simulink model "VFlexP"  (R2025a)
settings: Solver=ode23tb  StartTime=0.0  StopTime=40  FixedStep=5e-5
model workspace (MAT data in the model file):
  DCop_DCBUCK : object (value not decoded)
  Grid_CCVSC_idx = [2; 3; 4; 5; 6; 7; 8; 9; 10; 11; 12]
  Grid_CCVSCs = 1
  Grid_CCVSCs_buses = 1
  Grid_CCVSCs_toM = [0 1 0 0 0 0 0 0 0 0 0 0 ... (781 elements, 71x11)]
  Grid_C_Lines = [0.1 0.1 0.1 0.1]
  Grid_Cbuses = [0.05000002 0.10000002 0.10000002 0.10000002 0.05000002]
  Grid_DC : object (value not decoded)
  Grid_DCop_DCBUCK : object (value not decoded)
  Grid_DCop_DC_PES : object (value not decoded)
  Grid_DFIGs = 1
  Grid_DFIGs_buses = 1
  Grid_DGs : string (value not decoded)
  Grid_From_buses = [1 2 4 4]
  Grid_GFls = 1
  Grid_GFls_buses = 1
  Grid_GFr_idx = [1; 2; 3]
  Grid_GFrs = 1
  Grid_GFrs_buses = 1
  Grid_GFrs_toM = [1 0 0 0 0 0 0 0 0 1 0 0 ... (15 elements, 5x3)]
  Grid_IG_idx = 1
  Grid_IGs = 1
  Grid_IGs_buses = 1
  Grid_IGs_toM = [1; 0]
  Grid_L_Lines = [0.5 0.5 0.5 0.5]
  Grid_L_Loads = [0.000959999944704 0.000156249997559 0.00154855477548]
  Grid_Lines_fromM : object (value not decoded)
  Grid_Lines_toM : object (value not decoded)
  Grid_Load_buses = [2; 3; 4]
  Grid_Load_busesDC = []
  Grid_MGES_idx = [1; 2; 3]
  Grid_MGESs = 1
  Grid_MGESs_buses = [1; 5; 3]
  Grid_MGESs_toM = [1 0 0 0 0 0 0 0 0 1 0 0 ... (15 elements, 5x3)]
  Grid_MSGs = 1
  Grid_MSGs_buses = 1
  Grid_Nbuses = 5
  Grid_PQ_gen = [3; 2; 2]
  Grid_Ploads = [1250 4000 1250]
  Grid_PloadsDC = []
  Grid_Ps_lf = [0.274439537683 0.78 0.3]
  Grid_Qloads = [0.3 0.5 0.5]
  Grid_Qs_lf = [-0.0366071562958 0.126505596722 -0.0162964024532]
  Grid_R_Lines = [0.01 0.01 0.01 0.01]
  Grid_R_Loads = [3.9999997696 1.24999998047 3.8713869387]
  Grid_R_Loads_DC = 0
  Grid_Rcf = [50000000 50000000 50000000 50000000 50000000]
  Grid_SCs = 1
  Grid_SCs_buses = 1
  Grid_SG_idx = 1
  Grid_SGs = 1
  Grid_SGs_buses = 1
  Grid_SGs_toM = [1; 0]
  Grid_To_buses = [2 3 3 5]
  Grid_VCVSC_idx = [1; 2; 3; 4; 5; 6; 7; 8; 9; 10; 11; 12]
  Grid_VCVSCs = 1
  Grid_VCVSCs_buses = [1; 2; 3; 6; 8; 9; 12; 58; 59; 60; 63; 65]
  Grid_VCVSCs_toM = [1 0 0 0 0 0 0 0 0 0 0 0 ... (852 elements, 71x12)]
  Grid_VSM_idx = [1; 2; 3]
  Grid_VSMs = 1
  Grid_VSMs_buses = 1
  Grid_VSMs_toM = [1 0 0 0 0 0 0 0 0 1 0 0 ... (15 elements, 5x3)]
  Grid_admitt_matrix = [2.15353135314-19.7953135314i  -1.9801980198+19.801980198i; -1.9801980198+19.801980198i  2.15353135314-19.7953135314i]
  Grid_admitt_matrix_noloads = [1.98686468647-19.7953135314i  -1.9801980198+19.801980198i; -1.9801980198+19.801980198i  1.98686468647-19.7953135314i]
  Grid_bus = [1; 2; 6; 7; 8]
  Grid_busDC_complexity = [1 1 1]
  Grid_busDC_complexity_PF = [2 2 2]
  Grid_bus_complexity = [1 1 1 1 1]
  Grid_bus_complexity_PF = [1 1 1 1 1]
  Grid_buses_lf = [1; 5; 3]
  Grid_conductance_matrix = [100.00000002  -100  0; -100  200.00000002  -100; 0  -100  100.00000002]
  Grid_conductance_matrix_noloads = [100.00000002  -100  0; -100  200.00000002  -100; 0  -100  100.00000002]
  Grid_fref : object (value not decoded)
  Grid_gen_static_params : mBase (value not decoded)
  Grid_iPs_lf = [3.64378984326 1.28205128205 3.33333333333]
  Grid_iQs_lf = [-27.3170631425 7.90478860943 -61.3632366329]
  Grid_iadmitt_matrix = [2.88165849328-0.0982918688642i  2.87905051706-0.123273862303i; 2.87905051706-0.123273862303i  2.88165849328-0.0982918688642i]
  Grid_iadmitt_matrix_noloads = [37.5012524798-37.4874983544i  37.4987475202-37.5125016456i; 37.4987475202-37.5125016456i  37.5012524798-37.4874983544i]
  Grid_iconductance_matrix = [16666671.4556  16666671.4489  16666671.4456; 16666671.4489  16666671.4522  16666671.4489; 16666671.4456  16666671.4489  16666671.4556]
  Grid_iconductance_matrix_noloads = [16666671.4556  16666671.4489  16666671.4456; 16666671.4489  16666671.4522  16666671.4489; 16666671.4456  16666671.4489  16666671.4556]
  Grid_init_OK_bool = 1
  Grid_intconv_PF : object (value not decoded)
  Grid_lf_op : op_report (value not decoded)
  Grid_lineDC_complexity = [1 1]
  Grid_lineDC_complexity_PF = [2 2]
  Grid_line_complexity = [1 1 1 1]
  Grid_line_complexity_PF = [3 3 3 3]
  Grid_loadDC_complexity = []
  Grid_loadDC_complexity_PF = []
  Grid_load_complexity = [3 3 3]
  Grid_load_complexity_PF = [4 4 4]
  Grid_opDC_CCVSC : object (value not decoded)
  Grid_opDC_VSM : object (value not decoded)
  Grid_opGFr : object (value not decoded)
  Grid_opVCVSC : object (value not decoded)
  Grid_op_CCVSC : object (value not decoded)
  Grid_op_IG : object (value not decoded)
  Grid_op_MGES : object (value not decoded)
  Grid_op_SG : object (value not decoded)
  Grid_op_VSM : object (value not decoded)
  Grid_shift_lines = [0 0 0 0]
  Grid_tap_lines = [1 1 1 1]
  Grid_v_buses_mod = [1 1 1 0.9837920967 1]
  LinsysParamChangeStruct : Param1 (value not decoded)
  Lline = 0.01
  Rline = 1e-05
  linsys : object (value not decoded)
symbols that are objects in the model workspace (value not decoded): Grid_DCop_DC_PES, Grid_DCop_DCBUCK, Grid_op_CCVSC, Grid_op_IG, Grid_op_MGES, Grid_op_SG, Grid_op_VSM, Grid_opDC_CCVSC, Grid_opDC_VSM, Grid_opGFr, Grid_opVCVSC
undefined symbols (not defined in the file): block_buses_DC, block_idx, CCVSC_idx, Cf, costs, costs2, D, DFIGs_nodes, DiscIntNeverNeededParam, entity, Fb, Fi, From_nodes, grid_linsys, Grid_op_DFIG, Grid_op_DFIG_PQ, Grid_op_MSG, Grid_op_SC, Grid_op_VCVSC, H, initial_states_grid, K_1, K_3, K_5, K_A, K_C, K_IM, K_IR, K_P, K_PM, K_PR, K_S1, K_S2, K_S3, Ki_w, Kic, Kiv, Kp_id, Kp_theta, Kp_w, Kpc, Kpv, last_send, Lc, Lf, Lfd, Lkd1, Lkd2, Lkq1, Lkq2, Lkq3, Lmd, Lmq, Lsd, Lsq, m, M, Matrix_flux_to_i, mp, MSGs_buses ... (+44)
libraries: simulink x1048, eeGeneralControl x12
(part 26 of 50)

== system VFlexP/Grid/DCAC converters/DC_VCVSC/RL out/dynamic ==
  v_in_d : Inport
  v_out_d : Inport  Port=2
  v_in_q : Inport  Port=3
  v_out_q : Inport  Port=4
  Gain1 : Gain  Gain=L
  Gain2 : Gain  Gain=R
  Gain3 : Gain  Gain=R
  Gain4 : Gain  Gain=L
  Gain5 : Gain  Gain=invL*omegab
  Gain7 : Gain  Gain=invL*omegab
  Product : Product
  Product1 : Product
  Sum4 : Sum  Inputs=+-|
  Sum5 : Sum  Inputs=|-+
  Sum6 : Sum  Inputs=|++
  Sum7 : Sum  Inputs=-+|
  Sum8 : Sum  Inputs=|+-
  Sum9 : Sum  Inputs=-+|
  i_d : Integrator  InitialCondition=Grid_op_VCVSC.States(9,:)
  i_q : Integrator  InitialCondition=Grid_op_VCVSC.States(10,:)
  id : Outport
  iq : Outport  Port=2
  v_outd : Outport  Port=3
  v_outq : Outport  Port=4
  wires:
  v_in_q/1 -> Sum5/2  "v_in_q"
  v_in_d/1 -> Sum4/1  "v_in_d"
  Gain2/1 -> Sum4/2
  i_d/1 -> Gain2/1, Gain1/1, id/1  "id"
  Sum6/1 -> Gain5/1
  [omega_ref] -> Product1/1, Product/2  "omega"
  Gain5/1 -> i_d/1
  Product/1 -> Sum6/2
  Sum8/1 -> Gain7/1
  Sum4/1 -> Sum7/2
  Product1/1 -> Sum8/2
  Gain4/1 -> Product/1
  Sum7/1 -> Sum6/1
  Gain3/1 -> Sum5/1
  Sum5/1 -> Sum9/2
  Gain7/1 -> i_q/1
  i_q/1 -> Gain3/1, Gain4/1, iq/1  "iq"
  Gain1/1 -> Product1/2
  Sum9/1 -> Sum8/1
  v_out_d/1 -> Sum7/1, v_outd/1  "v_out_d"
  v_out_q/1 -> Sum9/1, v_outq/1  "v_out_q"

== system VFlexP/Grid/DCAC converters/DC_VCVSC/RL out/static ==
  v_in_d : Inport
  v_out_d : Inport  Port=2
  v_in_q : Inport  Port=3
  v_out_q : Inport  Port=4
  Constant : Constant  Value=R.^2
  Constant1 : Constant
  Divide : Product  Inputs=*/
  Gain : Gain  Gain=L
  Gain1 : Gain  Gain=R
  Gain2 : Gain  Gain=R
  Product{,1..5} (6 alike) : Product
  Sum : Sum  Inputs=|++
  Sum1 : Sum  Inputs=|+-
  Sum2 : Sum  Inputs=|+-
  Sum3 : Sum  Inputs=|++
  Sum4 : Sum  Inputs=|-+
  id : Outport
  iq : Outport  Port=2
  v_outd : Outport  Port=3
  v_outq : Outport  Port=4
  wires:
  v_in_q/1 -> Sum2/1  "v_in_q"
  v_out_d/1 -> Sum1/2, v_outd/1  "v_out_d"
  Sum/1 -> Divide/2
  Gain2/1 -> Product5/2
  Product/1 -> Sum/2
  Product1/1 -> Sum3/1
  Product5/1 -> Sum4/2
  Constant/1 -> Sum/1
  Sum2/1 -> Product3/2, Product5/1  "vq"
  Gain/1 -> Product2/2, Product/1, Product/2
  Constant1/1 -> Divide/1
  Product3/1 -> Sum3/2
  Sum1/1 -> Product4/1, Product1/1  "vd"
  Divide/1 -> Product2/1, Gain1/1, Gain2/1
  Product4/1 -> Sum4/1
  Product2/1 -> Product3/1, Product4/2
  Gain1/1 -> Product1/2
  Sum3/1 -> id/1  "id"
  Sum4/1 -> iq/1  "iq"
  v_out_q/1 -> Sum2/2, v_outq/1  "v_out_q"
  v_in_d/1 -> Sum1/1  "v_in_d"
  [omega_ref] -> Gain/1  "omega"

== system VFlexP/Grid/DCAC converters/DC_VCVSC/RL out/static_omega ==
  v_in_d : Inport
  v_out_d : Inport  Port=2
  v_in_q : Inport  Port=3
  v_out_q : Inport  Port=4
  Gain : Gain  Gain=1./(R.^2+L.^2)
  Gain2 : Gain  Gain=1./(R.^2+L.^2)
  Gain3 : Gain  Gain=R
  Gain4 : Gain  Gain=L
  Gain5 : Gain  Gain=L
  Gain6 : Gain  Gain=R
  Sum : Sum  Inputs=|++
  Sum1 : Sum  Inputs=|+-
  Sum2 : Sum  Inputs=|+-
  Sum3 : Sum  Inputs=|-+
  id : Outport
  iq : Outport  Port=2
  v_outd : Outport  Port=3
  v_outq : Outport  Port=4
  wires:
  Gain6/1 -> Sum3/2
  Sum3/1 -> iq/1
  Gain5/1 -> Sum3/1
  Sum/1 -> id/1
  Gain2/1 -> Gain4/1, Gain6/1
  Gain4/1 -> Sum/2
  Gain3/1 -> Sum/1
  Gain/1 -> Gain3/1, Gain5/1
  Sum2/1 -> Gain2/1  "vq"
  Sum1/1 -> Gain/1  "vd"
  v_out_d/1 -> Sum1/2, v_outd/1  "v_out_d"
  v_out_q/1 -> Sum2/2, v_outq/1  "v_out_q"
  v_in_d/1 -> Sum1/1  "v_in_d"
  v_in_q/1 -> Sum2/1  "v_in_q"

== system VFlexP/Grid/DCAC converters/DC_VCVSC/VCC/dynamic ==
  vodref : Inport
  voqref : Inport  Port=2
  iod : Inport  Port=3
  ioq : Inport  Port=4
  omega : Inport  Port=5
  Cf : Gain  Gain=Cfi
  Cf 1 : Gain  Gain=Cfi
  Fi : Gain  Gain=Fi
  Fi2 : Gain  Gain=Fi
  "Lf " : Gain  Gain=Lf
  Lf1 : Gain  Gain=Lf
  Product{,1..3} (4 alike) : Product
  RC : Subsystem  Variant=on  VariantControlMode=label  LabelModeActiveChoice=dynamic  mask{dynamic=Dynamic, R=Rcf, C=Cfi, fbase=50}
      mask prompts: dynamic "Dynamic behavior"; R "Parallel resistance (p.u.)"; C "Capacitance (p.u.)"; fbase "Base frequency (Hz)"
      mask init:
      | omegab = 2*pi*fbase;
      | iC = 1./C;
      | iR = 1./R;
      | vssBlk = gcb;
      | switch dynamic
      |     case "Dynamic"
      |         set_param(vssBlk, 'LabelModeActiveChoice', 'dynamic');
      |     case "Static"
      |         set_param(vssBlk, 'LabelModeActiveChoice', 'static');
      |     case "Static omega"
      |         set_param(vssBlk, 'LabelModeActiveChoice', 'static omega');
      | end
      mask TypeOptions dynamic: Dynamic | Static | Static omega
  RL : Subsystem  Variant=on  VariantControlMode=label  LabelModeActiveChoice=dynamic  mask(Line){dynamic=Dynamic, R=Rf, L=Lf, fbase=fb}
      mask prompts: dynamic "Dynamic behavior"; R "Series resistance (p.u.)"; L "Inductance (p.u.)"; fbase "Base frequency (Hz)"
      mask init: same as VFlexP/Grid/DCAC converters/DC_VCVSC/RL out
      mask Help: web('Documentation/RL.html')
      mask TypeOptions dynamic: Static | Dynamic | Static omega
  Subsystem : Subsystem
  Subsystem1 : Subsystem
  Subsystem2 : Subsystem
  Subsystem3 : Subsystem
  Sum1 : Sum  Inputs=++|
  Sum2 : Sum  Inputs=-+|
  Sum{3,5..6,9} (4 alike) : Sum  Inputs=|++
  Sum4 : Sum  Inputs=++|
  Sum8 : Sum  Inputs=-+|
  vidref : Outport
  viqref : Outport  Port=2
  wires:
  Sum6/1 -> RL/3(v_in_q)
  Sum1/1 -> RL/1(v_in_d)
  Sum9/1 -> Sum6/1  "viqref"
  Sum8/1 -> Sum1/2  "vidref"
  RL/2(iq) -> "Lf "/1, Subsystem3/2(y), RC/3(i_q_in)
  RL/1(id) -> RC/1(i_d_in), Lf1/1, Subsystem2/2(y)
  RC/1(v_d) -> Cf 1/1, Subsystem/2(y), RL/2(v_out_d), Sum1/1, vidref/1
  [omega] -> Product1/1
  omega/1 -> [omega], Product2/1  "omega"
  Subsystem3/1(Out1) -> Sum9/1
  Subsystem2/1(Out1) -> Sum8/2
  Subsystem1/1(Out1) -> Sum3/1
  Subsystem/1(Out1) -> Sum2/2
  Fi2/1 -> Sum5/2
  ioq/1 -> Fi2/1, RC/4(i_q_out)  "ioq"
  [omega] -> Product3/1, RC/5(omega)  "omega"
  Sum3/1 -> Sum5/1
  "Lf "/1 -> Product/1
  Sum2/1 -> Sum4/2
  iod/1 -> Fi/1, RC/2(i_d_out)  "iod"
  Product1/1 -> Sum2/1
  Sum4/1 -> Subsystem2/1(ref)  "ildref"
  Cf/1 -> Product1/2
  Cf 1/1 -> Product2/2
  Product2/1 -> Sum3/2
  Product3/1 -> Sum9/2
  voqref/1 -> Subsystem1/1(ref)  "voqref"
  Fi/1 -> Sum4/1
  Lf1/1 -> Product3/2
  [omega] -> Product/2
  RC/2(v_q) -> Cf/1, Subsystem1/2(y), RL/4(v_out_q), Sum6/2, viqref/1  "voq"
  vodref/1 -> Subsystem/1(ref)  "vodref"
  Product/1 -> Sum8/1
  Sum5/1 -> Subsystem3/1(ref)  "ilqref"

== system VFlexP/Grid/DCAC converters/DC_VCVSC/VCC/dynamic_VC ==
  vodref : Inport
  voqref : Inport  Port=2
  iod : Inport  Port=3
  ioq : Inport  Port=4
  omega : Inport  Port=5
  Cf : Gain  Gain=Cfi
  Cf 1 : Gain  Gain=Cfi
  Fi : Gain  Gain=Fi
  Fi2 : Gain  Gain=Fi
  Product1 : Product
  Product2 : Product
  RC : Subsystem  Variant=on  VariantControlMode=label  LabelModeActiveChoice=dynamic  mask{dynamic=Dynamic, R=Rcf, C=Cfi, fbase=50}
      mask prompts: dynamic "Dynamic behavior"; R "Parallel resistance (p.u.)"; C "Capacitance (p.u.)"; fbase "Base frequency (Hz)"
      mask init: same as VFlexP/Grid/DCAC converters/DC_VCVSC/VCC/dynamic/RC
      mask TypeOptions dynamic: Dynamic | Static | Static omega
  Subsystem : Subsystem
  Subsystem1 : Subsystem
  Sum2 : Sum  Inputs=-+|
  Sum3 : Sum  Inputs=|++
  Sum4 : Sum  Inputs=++|
  Sum5 : Sum  Inputs=|++
  vidref : Outport
  viqref : Outport  Port=2
  wires:
  Sum5/1 -> RC/3(i_q_in)
  Sum4/1 -> RC/1(i_d_in)
  RC/1(v_d) -> Subsystem/2(y), Cf 1/1, vidref/1
  vodref/1 -> Subsystem/1(ref)  "vodref"
  RC/2(v_q) -> Subsystem1/2(y), Cf/1, viqref/1
  Fi/1 -> Sum4/1
  voqref/1 -> Subsystem1/1(ref)  "voqref"
  Product2/1 -> Sum3/2
  Cf 1/1 -> Product2/2
  Cf/1 -> Product1/2
  Product1/1 -> Sum2/1
  iod/1 -> Fi/1, RC/2(i_d_out)  "iod"
  Sum2/1 -> Sum4/2
  Sum3/1 -> Sum5/1
  ioq/1 -> Fi2/1, RC/4(i_q_out)  "ioq"
  Fi2/1 -> Sum5/2
  Subsystem/1(Out1) -> Sum2/2
  Subsystem1/1(Out1) -> Sum3/1
  omega/1 -> [omega], Product2/1, RC/5(omega)  "omega"
  [omega] -> Product1/1

== system VFlexP/Grid/DCAC converters/DC_VCVSC/VCC/dynamic_limiting ==
  note: Current limiting, no priority
  vodref : Inport
  voqref : Inport  Port=2
  iod : Inport  Port=3
  ioq : Inport  Port=4
  omega : Inport  Port=5
  Abs : Abs  ZeroCross=off  SaturateOnIntegerOverflow=off
  Abs1 : Abs  ZeroCross=off  SaturateOnIntegerOverflow=off
  Abs2 : Abs  ZeroCross=off  SaturateOnIntegerOverflow=off
  Cf : Gain  Gain=Cfi
  Cf 1 : Gain  Gain=Cfi
  Divide : Product  Inputs=*/
  Divide1 : Product  Inputs=*/
  Fi : Gain  Gain=Fi
  Fi2 : Gain  Gain=Fi
  Gain : Gain  Gain=-1
  Gain1 : Gain  Gain=-1
  "Lf " : Gain  Gain=Lf
  Lf1 : Gain  Gain=Lf
  Memory : Memory  InitialCondition=1  LinearizeMemory=on
  Memory1 : Memory  InitialCondition=1  LinearizeMemory=on
  PIi_d : Subsystem
  PIi_q : Subsystem
  PIv_d : Subsystem
  PIv_q : Subsystem
  Product{,1..3} (4 alike) : Product
  RC : Subsystem  Variant=on  VariantControlMode=label  LabelModeActiveChoice=dynamic  mask{dynamic=Dynamic, R=Rcf, C=Cfi, fbase=50}
      mask prompts: dynamic "Dynamic behavior"; R "Parallel resistance (p.u.)"; C "Capacitance (p.u.)"; fbase "Base frequency (Hz)"
      mask init: same as VFlexP/Grid/DCAC converters/DC_VCVSC/VCC/dynamic/RC
      mask TypeOptions dynamic: Dynamic | Static | Static omega
  RL : Subsystem  Variant=on  VariantControlMode=label  LabelModeActiveChoice=dynamic  mask(Line){dynamic=Dynamic, R=Rf, L=Lf, fbase=fb}
      mask prompts: dynamic "Dynamic behavior"; R "Series resistance (p.u.)"; L "Inductance (p.u.)"; fbase "Base frequency (Hz)"
      mask init: same as VFlexP/Grid/DCAC converters/DC_VCVSC/RL out
      mask Help: web('Documentation/RL.html')
      mask TypeOptions dynamic: Static | Dynamic | Static omega
  Real-Imag to Complex : RealImagToComplex
  Relational Operator : RelationalOperator  Operator===  OutDataTypeStr=boolean  ZeroCross=off  RndMeth=Simplest  InputSameDT=off
  Relational Operator1 : RelationalOperator  Operator===  OutDataTypeStr=boolean  ZeroCross=off  RndMeth=Simplest  InputSameDT=off
  Saturation Dynamic : simulink/Discontinuities/Saturation Dynamic  OutMin=[]  OutMax=[]  OutDataTypeStr=Inherit: Same as second input  OutDataType=fixdt(1, 16)  OutScaling=2^-10  DoSatur=off
  Saturation Dynamic1 : simulink/Discontinuities/Saturation Dynamic  OutMin=[]  OutMax=[]  OutDataTypeStr=Inherit: Same as second input  OutDataType=fixdt(1, 16)  OutScaling=2^-10  DoSatur=off
  Sum : Sum  Inputs=|+-
  Sum{1..2,6,8} (4 alike) : Sum  Inputs=-+|
  Sum3 : Sum  Inputs=|++
  Sum4 : Sum  Inputs=++|
  Sum5 : Sum  Inputs=|++
  Sum7 : Sum  Inputs=|+-
  Sum9 : Sum  Inputs=|++
  vidref : Outport
  viqref : Outport  Port=2
  wires:
  Memory/1 -> PIv_d/2(In2)
  Memory1/1 -> PIv_q/2(In2)
  Relational Operator1/1 -> Memory1/1
  Sum/1 -> PIv_q/1(In1)
  Relational Operator/1 -> Memory/1
  Sum1/1 -> PIv_d/1(In1)
  Gain1/1 -> Saturation Dynamic/3
  Gain/1 -> Saturation Dynamic1/3
  Divide1/1 -> Saturation Dynamic1/1, Gain/1
  Divide/1 -> Saturation Dynamic/1, Gain1/1
  Abs/1 -> Divide/2, Divide1/2
  Real-Imag to Complex/1 -> Abs/1
  Sum5/1 -> Real-Imag to Complex/2, Saturation Dynamic1/2, Abs1/1, Relational Operator1/1  "ilqref"
  Product/1 -> Sum8/1
  vodref/1 -> Sum1/2  "vodref"
  RC/2(v_q) -> viqref/1, RL/4(v_out_q), Sum/2, Cf/1  "voq"
  [omega] -> Product/2
  Lf1/1 -> Product3/2
  Fi/1 -> Sum4/1
  Sum6/1 -> PIi_d/1(In1)
  voqref/1 -> Sum/1  "voqref"
  Product3/1 -> Sum9/2
  Product2/1 -> Sum3/2
  Cf 1/1 -> Product2/2
  Cf/1 -> Product1/2
  Sum4/1 -> Real-Imag to Complex/1, Saturation Dynamic/2, Abs2/1, Relational Operator/1  "ildref"
  Product1/1 -> Sum2/1
  iod/1 -> RC/2(i_d_out), Fi/1  "iod"
  Sum2/1 -> Sum4/2
  Sum7/1 -> PIi_q/1(In1)
  "Lf "/1 -> Product/1
  Sum3/1 -> Sum5/1
  [omega] -> RC/5(omega), Product3/1  "omega"
  ioq/1 -> RC/4(i_q_out), Fi2/1  "ioq"
  Fi2/1 -> Sum5/2
  PIv_d/1(Out1) -> Sum2/2
  PIv_q/1(Out1) -> Sum3/1
  PIi_d/1(Out1) -> Sum8/2
  PIi_q/1(Out1) -> Sum9/1
  omega/1 -> Product2/1, [omega]  "omega"
  [omega] -> Product1/1
  RC/1(v_d) -> vidref/1, RL/2(v_out_d), Cf 1/1, Sum1/1
  RL/1(id) -> Lf1/1, Sum6/1, RC/1(i_d_in)
  RL/2(iq) -> RC/3(i_q_in), "Lf "/1, Sum7/2
  Sum8/1 -> RL/1(v_in_d)  "vidref"
  Sum9/1 -> RL/3(v_in_q)  "viqref"
  Abs1/1 -> Divide1/1
  Abs2/1 -> Divide/1
  Saturation Dynamic1/1 -> Relational Operator1/2, Sum7/1
  Saturation Dynamic/1 -> Relational Operator/2, Sum6/2

== system VFlexP/Grid/DCAC converters/DC_VCVSC/VCC/static ==
  vodref : Inport
  voqref : Inport  Port=2
  iod : Inport  Port=3
  ioq : Inport  Port=4
  omega : Inport  Port=5
  Terminator : Terminator
  Terminator1 : Terminator
  Terminator2 : Terminator
  vidref : Outport
  viqref : Outport  Port=2
  wires:
  omega/1 -> Terminator2/1  "ioq"
  ioq/1 -> Terminator1/1  "ioq"
  iod/1 -> Terminator/1  "iod"
  vodref/1 -> vidref/1  "vodref"
  voqref/1 -> viqref/1  "voqref"

== system VFlexP/Grid/DCAC converters/DC_VCVSC/VI/WOF_d ==
  In1 : Inport
  Gain : Gain  Gain=iTf
  I : Integrator  InitialConditionSource=external  InitialCondition=Grid_op_VCVSC.op.States(6).x'
  Sum : Sum  Inputs=+-|
  Sum4 : Sum  Inputs=|+-
  Out1 : Outport
  wires:
  Gain/1 -> I/1
  Sum4/1 -> Gain/1
  In1/1 -> I/2, Sum/1, Sum4/1
  I/1 -> Sum/2, Sum4/2
  Sum/1 -> Out1/1

== system VFlexP/Grid/DCAC converters/DC_VCVSC/VI/WOF_q ==
  In1 : Inport
  Gain : Gain  Gain=iTf
  I : Integrator  InitialConditionSource=external  InitialCondition=Grid_op_VCVSC.op.States(7).x'
  Sum : Sum  Inputs=+-|
  Sum4 : Sum  Inputs=|+-
  Out1 : Outport
  wires:
  Gain/1 -> I/1
  Sum4/1 -> Gain/1
  In1/1 -> I/2, Sum/1, Sum4/1
  I/1 -> Sum/2, Sum4/2
  Sum/1 -> Out1/1

== system VFlexP/Grid/DCAC converters/DC_VSM/PC/LPF_P ==
  P : Inport
  Gain : Gain  Gain=1e4
  I : Integrator  InitialCondition=Grid_opDC_VSM.P
  Sum4 : Sum  Inputs=|+-
  P_f : Outport
  wires:
  Gain/1 -> I/1
  Sum4/1 -> Gain/1
  P/1 -> Sum4/1
  I/1 -> P_f/1, Sum4/2

== system VFlexP/Grid/DCAC converters/DC_VSM/PC/LPF_P2 ==
  P : Inport
  Gain : Gain  Gain=1e4
  I : Integrator  InitialCondition=Grid_opDC_VSM.P
  Sum4 : Sum  Inputs=|+-
  P_f : Outport
  wires:
  I/1 -> Sum4/2, P_f/1
  P/1 -> Sum4/1
  Sum4/1 -> Gain/1
  Gain/1 -> I/1

== system VFlexP/Grid/DCAC converters/DC_VSM/PC/LPF_Q ==
  Q : Inport
  Gain : Gain  Gain=iTf
  I : Integrator
  Sum4 : Sum  Inputs=|+-
  Q_f : Outport
  wires:
  Gain/1 -> I/1
  Q/1 -> Sum4/1
  I/1 -> Q_f/1, Sum4/2
  Sum4/1 -> Gain/1

== system VFlexP/Grid/DCAC converters/DC_VSM/PC/LPF_Q1 ==
  Q : Inport
  Gain : Gain  Gain=iTf
  I : Integrator  InitialConditionSource=external
  Sum4 : Sum  Inputs=|+-
  Q_f : Outport
  wires:
  Sum4/1 -> Gain/1
  I/1 -> Sum4/2, Q_f/1
  Q/1 -> I/2, Sum4/1
  Gain/1 -> I/1

== system VFlexP/Grid/DCAC converters/DC_VSM/PC/Turbine model ==
  In1 : Inport
  Out1 : Outport
  wires:
  In1/1 -> Out1/1

== system VFlexP/Grid/DCAC converters/DC_VSM/PC/WOF_d ==
  In1 : Inport
  Gain : Gain  Gain=10
  Gain1 : Gain  Gain=10
  I : Integrator  InitialConditionSource=external  InitialCondition=Grid_op_VSM.op.States(7).x'
  Sum : Sum  Inputs=+-|
  Sum4 : Sum  Inputs=|+-
  Out1 : Outport
  wires:
  Gain/1 -> I/1
  Sum4/1 -> Gain/1
  In1/1 -> I/2, Sum/1, Sum4/1
  I/1 -> Sum/2, Sum4/2
  Sum/1 -> Gain1/1
  Gain1/1 -> Out1/1

== system VFlexP/Grid/DCAC converters/DC_VSM/RL out/dynamic ==
  v_in_d : Inport
  v_out_d : Inport  Port=2
  v_in_q : Inport  Port=3
  v_out_q : Inport  Port=4
  Gain1 : Gain  Gain=L
  Gain2 : Gain  Gain=R
  Gain3 : Gain  Gain=R
  Gain4 : Gain  Gain=L
  Gain5 : Gain  Gain=invL*omegab
  Gain7 : Gain  Gain=invL*omegab
  Product : Product
  Product1 : Product
  Sum4 : Sum  Inputs=+-|
  Sum5 : Sum  Inputs=|-+
  Sum6 : Sum  Inputs=|++
  Sum7 : Sum  Inputs=-+|
  Sum8 : Sum  Inputs=|+-
  Sum9 : Sum  Inputs=-+|
  i_d : Integrator  InitialCondition=Grid_opDC_VSM.id_out
  i_q : Integrator  InitialCondition=Grid_opDC_VSM.iq_out
  id : Outport
  iq : Outport  Port=2
  v_outd : Outport  Port=3
  v_outq : Outport  Port=4
  wires:
  v_out_q/1 -> v_outq/1, Sum9/1  "v_out_q"
  v_out_d/1 -> v_outd/1, Sum7/1  "v_out_d"
  Sum9/1 -> Sum8/1
  Gain1/1 -> Product1/2
  i_q/1 -> iq/1, Gain4/1, Gain3/1  "iq"
  Gain7/1 -> i_q/1
  Sum5/1 -> Sum9/2
  Gain3/1 -> Sum5/1
  Sum7/1 -> Sum6/1
  Gain4/1 -> Product/1
  Product1/1 -> Sum8/2
  Sum4/1 -> Sum7/2
  Sum8/1 -> Gain7/1
  Product/1 -> Sum6/2
  Gain5/1 -> i_d/1
  [omega_ref] -> Product/2, Product1/1  "omega"
  Sum6/1 -> Gain5/1
  i_d/1 -> id/1, Gain1/1, Gain2/1  "id"
  Gain2/1 -> Sum4/2
  v_in_d/1 -> Sum4/1  "v_in_d"
  v_in_q/1 -> Sum5/2  "v_in_q"

== system VFlexP/Grid/DCAC converters/DC_VSM/RL out/static ==
  v_in_d : Inport
  v_out_d : Inport  Port=2
  v_in_q : Inport  Port=3
  v_out_q : Inport  Port=4
  Constant : Constant  Value=R.^2
  Constant1 : Constant
  Divide : Product  Inputs=*/
  Gain : Gain  Gain=L
  Gain1 : Gain  Gain=R
  Gain2 : Gain  Gain=R
  Product{,1..5} (6 alike) : Product
  Sum : Sum  Inputs=|++
  Sum1 : Sum  Inputs=|+-
  Sum2 : Sum  Inputs=|+-
  Sum3 : Sum  Inputs=|++
  Sum4 : Sum  Inputs=|-+
  id : Outport
  iq : Outport  Port=2
  v_outd : Outport  Port=3
  v_outq : Outport  Port=4
  wires:
  [omega_ref] -> Gain/1  "omega"
  v_in_d/1 -> Sum1/1  "v_in_d"
  v_out_q/1 -> v_outq/1, Sum2/2  "v_out_q"
  Sum4/1 -> iq/1  "iq"
  Sum3/1 -> id/1  "id"
  Gain1/1 -> Product1/2
  Product2/1 -> Product4/2, Product3/1
  Product4/1 -> Sum4/1
  Divide/1 -> Gain2/1, Gain1/1, Product2/1
  Sum1/1 -> Product1/1, Product4/1  "vd"
  Product3/1 -> Sum3/2
  Constant1/1 -> Divide/1
  Gain/1 -> Product/2, Product/1, Product2/2
  Sum2/1 -> Product5/1, Product3/2  "vq"
  Constant/1 -> Sum/1
  Product5/1 -> Sum4/2
  Product1/1 -> Sum3/1
  Product/1 -> Sum/2
  Gain2/1 -> Product5/2
  Sum/1 -> Divide/2
  v_out_d/1 -> v_outd/1, Sum1/2  "v_out_d"
  v_in_q/1 -> Sum2/1  "v_in_q"

== system VFlexP/Grid/DCAC converters/DC_VSM/RL out/static_omega ==
  v_in_d : Inport
  v_out_d : Inport  Port=2
  v_in_q : Inport  Port=3
  v_out_q : Inport  Port=4
  Gain : Gain  Gain=1./(R.^2+L.^2)
  Gain2 : Gain  Gain=1./(R.^2+L.^2)
  Gain3 : Gain  Gain=R
  Gain4 : Gain  Gain=L
  Gain5 : Gain  Gain=L
  Gain6 : Gain  Gain=R
  Sum : Sum  Inputs=|++
  Sum1 : Sum  Inputs=|+-
  Sum2 : Sum  Inputs=|+-
  Sum3 : Sum  Inputs=|-+
  id : Outport
  iq : Outport  Port=2
  v_outd : Outport  Port=3
  v_outq : Outport  Port=4
  wires:
  v_in_q/1 -> Sum2/1  "v_in_q"
  v_in_d/1 -> Sum1/1  "v_in_d"
  v_out_q/1 -> v_outq/1, Sum2/2  "v_out_q"
  v_out_d/1 -> v_outd/1, Sum1/2  "v_out_d"
  Sum1/1 -> Gain/1  "vd"
  Sum2/1 -> Gain2/1  "vq"
  Gain/1 -> Gain5/1, Gain3/1
  Gain3/1 -> Sum/1
  Gain4/1 -> Sum/2
  Gain2/1 -> Gain6/1, Gain4/1
  Sum/1 -> id/1
  Gain5/1 -> Sum3/1
  Sum3/1 -> iq/1
  Gain6/1 -> Sum3/2

== system VFlexP/Grid/DCAC converters/DC_VSM/VCC/dynamic ==
  vodref : Inport
  voqref : Inport  Port=2
  iod : Inport  Port=3
  ioq : Inport  Port=4
  omega : Inport  Port=5
  Cf : Gain  Gain=Cfi
  Cf 1 : Gain  Gain=Cfi
  Fi : Gain  Gain=Fi
  Fi2 : Gain  Gain=Fi
  "Lf " : Gain  Gain=Lf
  Lf1 : Gain  Gain=Lf
  PIid : Subsystem
  PIiq : Subsystem
  PIvd : Subsystem
  PIvq : Subsystem
  Product{,1..3} (4 alike) : Product
  RC : Subsystem  Variant=on  VariantControlMode=label  LabelModeActiveChoice=dynamic  mask{dynamic=Dynamic, R=Rcf, C=Cfi, fbase=50}
      mask prompts: dynamic "Dynamic behavior"; R "Parallel resistance (p.u.)"; C "Capacitance (p.u.)"; fbase "Base frequency (Hz)"
      mask init: same as VFlexP/Grid/DCAC converters/DC_VCVSC/VCC/dynamic/RC
      mask TypeOptions dynamic: Dynamic | Static | Static omega
  RL : Subsystem  Variant=on  VariantControlMode=label  LabelModeActiveChoice=dynamic  mask(Line){dynamic=Dynamic, R=Rf, L=Lf, fbase=fb}
      mask prompts: dynamic "Dynamic behavior"; R "Series resistance (p.u.)"; L "Inductance (p.u.)"; fbase "Base frequency (Hz)"
      mask init: same as VFlexP/Grid/DCAC converters/DC_VCVSC/RL out
      mask Help: web('Documentation/RL.html')
      mask TypeOptions dynamic: Static | Dynamic | Static omega
  Sum1 : Sum  Inputs=++|
  Sum2 : Sum  Inputs=-+|
  Sum{3,5..6,9} (4 alike) : Sum  Inputs=|++
  Sum4 : Sum  Inputs=++|
  Sum8 : Sum  Inputs=-+|
  vidref : Outport
  viqref : Outport  Port=2
  wires:
  Sum5/1 -> PIiq/1(ref)  "ilqref"
  Product/1 -> Sum8/1
  vodref/1 -> PIvd/1(ref)  "vodref"
  RC/2(vq) -> viqref/1, Sum6/2, RL/4(v_out_q), PIvq/2(y), Cf/1  "voq"
  [omega] -> Product/2
  Lf1/1 -> Product3/2
  Fi/1 -> Sum4/1
  voqref/1 -> PIvq/1(ref)  "voqref"
  Product3/1 -> Sum9/2
  Product2/1 -> Sum3/2
  Cf 1/1 -> Product2/2
  Cf/1 -> Product1/2
  Sum4/1 -> PIid/1(ref)  "ildref"
  Product1/1 -> Sum2/1
  iod/1 -> RC/2(i_d_out), Fi/1  "iod"
  Sum2/1 -> Sum4/2
  "Lf "/1 -> Product/1
  Sum3/1 -> Sum5/1
  [omega] -> RC/5(omega), Product3/1  "omega"
  ioq/1 -> RC/4(i_q_out), Fi2/1  "ioq"
  Fi2/1 -> Sum5/2
  PIvd/1(Out1) -> Sum2/2
  PIvq/1(Out1) -> Sum3/1
  PIid/1(Out1) -> Sum8/2
  PIiq/1(Out1) -> Sum9/1
  omega/1 -> Product2/1, [omega]  "omega"
  [omega] -> Product1/1
  RC/1(vd) -> vidref/1, Sum1/1, RL/2(v_out_d), PIvd/2(y), Cf 1/1
  RL/1(id) -> PIid/2(y), Lf1/1, RC/1(i_d_in)
  RL/2(iq) -> RC/3(i_q_in), PIiq/2(y), "Lf "/1
  Sum8/1 -> Sum1/2  "vidref"
  Sum9/1 -> Sum6/1  "viqref"
  Sum1/1 -> RL/1(v_in_d)
  Sum6/1 -> RL/3(v_in_q)

== system VFlexP/Grid/DCAC converters/DC_VSM/VCC/dynamic_VC ==
  vodref : Inport
  voqref : Inport  Port=2
  iod : Inport  Port=3
  ioq : Inport  Port=4
  omega : Inport  Port=5
  Cf : Gain  Gain=Cfi
  Cf 1 : Gain  Gain=Cfi
  Fi : Gain  Gain=Fi
  Fi2 : Gain  Gain=Fi
  Product1 : Product
  Product2 : Product
  RC : Subsystem  Variant=on  VariantControlMode=label  LabelModeActiveChoice=dynamic  mask{dynamic=Dynamic, R=Rcf, C=Cfi, fbase=50}
      mask prompts: dynamic "Dynamic behavior"; R "Parallel resistance (p.u.)"; C "Capacitance (p.u.)"; fbase "Base frequency (Hz)"
      mask init: same as VFlexP/Grid/DCAC converters/DC_VCVSC/VCC/dynamic/RC
      mask TypeOptions dynamic: Dynamic | Static | Static omega
  Subsystem : Subsystem
  Subsystem1 : Subsystem
  Sum2 : Sum  Inputs=-+|
  Sum3 : Sum  Inputs=|++
  Sum4 : Sum  Inputs=++|
  Sum5 : Sum  Inputs=|++
  vidref : Outport
  viqref : Outport  Port=2
  wires:
  [omega] -> Product1/1
  omega/1 -> RC/5(omega), Product2/1, [omega]  "omega"
  Subsystem1/1(Out1) -> Sum3/1
  Subsystem/1(Out1) -> Sum2/2
  Fi2/1 -> Sum5/2
  ioq/1 -> RC/4(i_q_out), Fi2/1  "ioq"
  Sum3/1 -> Sum5/1
  Sum2/1 -> Sum4/2
  iod/1 -> RC/2(i_d_out), Fi/1  "iod"
  Product1/1 -> Sum2/1
  Cf/1 -> Product1/2
  Cf 1/1 -> Product2/2
  Product2/1 -> Sum3/2
  voqref/1 -> Subsystem1/1(ref)  "voqref"
  Fi/1 -> Sum4/1
  RC/2(v_q) -> viqref/1, Cf/1, Subsystem1/2(y)
  vodref/1 -> Subsystem/1(ref)  "vodref"
  RC/1(v_d) -> vidref/1, Cf 1/1, Subsystem/2(y)
  Sum4/1 -> RC/1(i_d_in)
  Sum5/1 -> RC/3(i_q_in)

== system VFlexP/Grid/DCAC converters/DC_VSM/VCC/dynamic_limiting ==
  vodref : Inport
  voqref : Inport  Port=2
  iod : Inport  Port=3
  ioq : Inport  Port=4
  omega : Inport  Port=5
  Cf : Gain  Gain=Cfi
  Cf 1 : Gain  Gain=Cfi
  Complex to Magnitude-Angle2 : ComplexToMagnitudeAngle  Output=Magnitude
  Complex to Magnitude-Angle3 : ComplexToMagnitudeAngle
  Complex to Magnitude-Angle4 : ComplexToMagnitudeAngle  Output=Magnitude
  Complex to Magnitude-Angle5 : ComplexToMagnitudeAngle  Output=Magnitude
  Complex to Real-Imag1 : ComplexToRealImag
  Fi : Gain  Gain=Fi
  Fi2 : Gain  Gain=Fi
  "Lf " : Gain  Gain=Lf
  Lf1 : Gain  Gain=Lf
  Magnitude-Angle to Complex : MagnitudeAngleToComplex
  Memory : Memory
  NOT : Logic  Operator=NOT  IconShape=distinctive  AllPortsSameDT=off  OutDataTypeStr=boolean
  PIid : Subsystem
  PIiq : Subsystem
  PIvd : Subsystem
      settings: PortSchema="{\"entries\":[{\"content\":{\"sides\":[{\"content\":{\"connectorIds\":[\"In1\",\"In2\"]},\"type\":\"ConnectorPlacement.EquallySpacedRectSide\",\"uuid\":\"218efe14-094c-4cdd-8e62-ef6089c75bbd\"},{\"content\":{\"connectorIds\":[\"Out1\"],\"side\":\"RIGHT\"},\"type\":\"ConnectorPlacement.EquallySpacedRectSide\",\"uuid\":\"287e2a8a-062a-4519-a86c-f141c6982dac\"},{\"content\":{\"connectorIds\":[\"In3\"],\"side\":\"TOP\"},\"type\":\"ConnectorPlacement.EquallySpacedRectSide\",\"uuid\":\"e88fce21-908c-492a-b265-04b05ce94be8\"}]},\"type\":\"ConnectorPlacement.EquallySpacedConnector\",\"uuid\":\"5c149457-da6d-4223-b1cb-56365173b759\"}],\"packageUris\":[\"http://schema.mathworks.com/mf0/Connector/R2020b\"],\"version\":\"1.0\"}"
  PIvq : Subsystem
      settings: PortSchema="{\"entries\":[{\"content\":{\"sides\":[{\"content\":{\"connectorIds\":[\"In1\",\"In2\"]},\"type\":\"ConnectorPlacement.EquallySpacedRectSide\",\"uuid\":\"218efe14-094c-4cdd-8e62-ef6089c75bbd\"},{\"content\":{\"connectorIds\":[\"Out1\"],\"side\":\"RIGHT\"},\"type\":\"ConnectorPlacement.EquallySpacedRectSide\",\"uuid\":\"287e2a8a-062a-4519-a86c-f141c6982dac\"},{\"content\":{\"connectorIds\":[],\"side\":\"TOP\"},\"type\":\"ConnectorPlacement.EquallySpacedRectSide\",\"uuid\":\"e88fce21-908c-492a-b265-04b05ce94be8\"},{\"content\":{\"connectorIds\":[\"In3\"],\"side\":\"BOTTOM\"},\"type\":\"ConnectorPlacement.EquallySpacedRectSide\",\"uuid\":\"db964aea-37c6-4226-90b6-d177a6d2ab38\"}]},\"type\":\"ConnectorPlacement.EquallySpacedConnector\",\"uuid\":\"5c149457-da6d-4223-b1cb-56365173b759\"}],\"packageUris\":[\"http://schema.mathworks.com/mf0/Connector/R2020b\"],\"version\":\"1.0\"}"
  Product{,1..5} (6 alike) : Product
  RC : Subsystem  Variant=on  VariantControlMode=label  LabelModeActiveChoice=dynamic  mask{dynamic=Dynamic, R=Rcf, C=Cfi}
      mask prompts: dynamic "Dynamic behavior"; R "Parallel resistance (p.u.)"; C "Capacitance (p.u.)"
      mask init:
      | iC = 1./C;
      | iR = 1./R;
      | vssBlk = gcb;
      | switch dynamic
      |     case "Dynamic"
      |         set_param(vssBlk, 'LabelModeActiveChoice', 'dynamic');
      |     case "Static"
      |         set_param(vssBlk, 'LabelModeActiveChoice', 'static');
      |     case "Static omega"
      |         set_param(vssBlk, 'LabelModeActiveChoice', 'static omega');
      | end
      mask TypeOptions dynamic: Dynamic | Static | Static omega
  RL : Subsystem  Variant=on  VariantControlMode=label  LabelModeActiveChoice=dynamic  mask(Line){dynamic=Dynamic, R=Rf, L=Lf}
      mask prompts: dynamic "Dynamic behavior"; R "Series resistance (p.u.)"; L "Inductance (p.u.)"
      mask init: same as VFlexP/Grid/Generators/GFr/RL out
      mask Help: web('Documentation/RL.html')
      mask TypeOptions dynamic: Static | Dynamic | Static omega
  Real-Imag to Complex{2..5} (4 alike) : RealImagToComplex
  Relational Operator : RelationalOperator  Operator===  OutDataTypeStr=boolean  RndMeth=Simplest  InputSameDT=off
  Saturation : Saturate  UpperLimit=0.1  LowerLimit=0
  Scope{1,3,6..8} (5 alike) : Scope
      Scope1 settings: ActiveDisplayYMinimum=-0.06728  ActiveDisplayYMaximum=0.79818  DataLoggingVariableName=ScopeData2
      Scope3 settings: ActiveDisplayYMinimum=0.01769  ActiveDisplayYMaximum=0.10915
      Scope6 settings: ActiveDisplayYMinimum=0.03196  ActiveDisplayYMaximum=0.13112  DataLoggingVariableName=ScopeData2
      Scope7 settings: ActiveDisplayYMinimum=0.86043  ActiveDisplayYMaximum=1.1554  DataLoggingVariableName=ScopeData3
      Scope8 settings: ActiveDisplayYMinimum=0.0318  ActiveDisplayYMaximum=0.12782  DataLoggingVariableName=ScopeData4
  Scope2 : Scope  NumInputPorts=2
      settings: ActiveDisplayYMinimum=-0.10019  ActiveDisplayYMaximum=0.20176
  Scope4 : Scope  NumInputPorts=2
      settings: ActiveDisplayYMinimum=-0.04364  ActiveDisplayYMaximum=0.0791  DataLoggingVariableName=ScopeData3
  Sum1 : Sum  Inputs=++|
  Sum{3,5..6,9,14..15} (6 alike) : Sum  Inputs=|++
  Sum2 : Sum  Inputs=-+|
  Sum4 : Sum  Inputs=++|
  Sum8 : Sum  Inputs=-+|
  VI : Subsystem  mask{L=0.5, R=0.1, Tf=0}
      mask prompts: L "Inductance (pu)"; R "Resistance (pu)"; Tf "WOF time constant (s)"
      mask init: same as VFlexP/Grid/DCAC converters/DC_VCVSC/VI
  vidref : Outport
  viqref : Outport  Port=2
  wires:
  Product/1 -> Sum8/1
  Sum14/1 -> PIvd/1(ref)  "vodref"
  RC/2(vq) -> [voq], viqref/1, RL/4(v_out_q), Sum6/2, PIvq/2(y), Cf/1, Real-Imag to Complex4/2  "voq"
  [omega] -> Product/2
  Lf1/1 -> Product3/2
  Fi/1 -> Sum4/1
  Sum15/1 -> PIvq/1(ref)  "voqref"
  Product3/1 -> Sum9/2
  Product2/1 -> Sum3/2
  Cf 1/1 -> Product2/2
  Cf/1 -> Product1/2
  Product1/1 -> Sum2/1
  iod/1 -> RC/2(i_d_out), Real-Imag to Complex5/1, Product4/2, Fi/1  "iod"
  Sum2/1 -> Sum4/2
  "Lf "/1 -> Product/1
  Sum3/1 -> Sum5/1
  [omega] -> RC/5(omega), RL/5(omega), Product3/1  "omega"
  ioq/1 -> RC/4(i_q_out), Fi2/1, Real-Imag to Complex5/2, Product5/2  "ioq"
  Fi2/1 -> Sum5/2
  PIvd/1(Out1) -> Sum2/2
  PIvq/1(Out1) -> Sum3/1
  PIid/1(Out1) -> Sum8/2
  PIiq/1(Out1) -> Sum9/1
  omega/1 -> Product2/1, [omega]  "omega"
  [omega] -> Product1/1
  RL/1(id) -> RC/1(i_d_in), Scope2/1, Real-Imag to Complex2/1, PIid/2(y), Lf1/1
  RL/2(iq) -> Scope4/1, PIiq/2(y), "Lf "/1, Real-Imag to Complex2/2, RC/3(i_q_in)
  Sum8/1 -> Sum1/2  "vidref"
  Sum9/1 -> Sum6/1  "viqref"
  Sum1/1 -> RL/1(v_in_d)
  Sum6/1 -> RL/3(v_in_q)
  Sum4/1 -> Real-Imag to Complex3/1, [ildref]  "ildref"
  Sum5/1 -> Real-Imag to Complex3/2, [ilqref]  "ilqref"
  RC/1(vd) -> Real-Imag to Complex4/1, RL/2(v_out_d), Sum1/1, [vod], vidref/1, PIvd/2(y), Cf 1/1
  Complex to Real-Imag1/2 -> Scope4/2, PIiq/1(ref)
  Real-Imag to Complex2/1 -> Complex to Magnitude-Angle2/1
  Complex to Magnitude-Angle2/1 -> Scope1/1  "i_mod"
  Complex to Real-Imag1/1 -> Scope2/2, PIid/1(ref)
  Real-Imag to Complex3/1 -> Complex to Magnitude-Angle3/1
  Saturation/1 -> Magnitude-Angle to Complex/1, Scope3/1, Relational Operator/1
  Relational Operator/1 -> PIvd/3(anti_windup), PIvq/3(anti_windup), NOT/1
  Complex to Magnitude-Angle3/1 -> Scope6/1, Relational Operator/2, Saturation/1
  Magnitude-Angle to Complex/1 -> Complex to Real-Imag1/1
  Complex to Magnitude-Angle3/2 -> Magnitude-Angle to Complex/2
  Complex to Magnitude-Angle4/1 -> Scope7/1  "vc_mod"
  Real-Imag to Complex4/1 -> Complex to Magnitude-Angle4/1
  Real-Imag to Complex5/1 -> Complex to Magnitude-Angle5/1
  Complex to Magnitude-Angle5/1 -> Scope8/1  "io_mod"
  vodref/1 -> Sum14/2  "vodref"
  voqref/1 -> Sum15/1  "voqref"
  NOT/1 -> Memory/1
  VI/1(vd) -> Sum14/1
  VI/2(vq) -> Sum15/2
  Memory/1 -> Product5/1, Product4/1
  Product4/1 -> VI/1(id)
  Product5/1 -> VI/2(iq)

== system VFlexP/Grid/DCAC converters/DC_VSM/VCC/dynamic_limiting_P ==
  vodref : Inport
  voqref : Inport  Port=2
  iod : Inport  Port=3
  ioq : Inport  Port=4
  omega : Inport  Port=5
  iP : Inport  Port=6
  Abs : Abs  SaturateOnIntegerOverflow=off
  Abs1 : Abs  SaturateOnIntegerOverflow=off
  Cf : Gain  Gain=Cfi
  Cf 1 : Gain  Gain=Cfi
  Complex to Magnitude-Angle : ComplexToMagnitudeAngle  Commented=on
  Complex to Magnitude-Angle5 : ComplexToMagnitudeAngle  Output=Magnitude
  Constant : Constant
  Constant2 : Constant  Commented=on  Value=Inf
  Dead Zone : DeadZone  LowerValue=-0.2  UpperValue=0.2
  Divide : Product  Commented=on  Inputs=*/
  Divide1 : Product  Inputs=*/
  Fi : Gain  Gain=Fi
  Fi2 : Gain  Gain=Fi
  From11 : From  Commented=on  GotoTag=ilqref
  From12 : From  Commented=on  GotoTag=ildref
  From13 : From  Commented=on  GotoTag=ildref
  From14 : From  Commented=on  GotoTag=ilqref
  From3 : From  Commented=on  GotoTag=vid
  From4 : From  Commented=on  GotoTag=viq
  Gain1 : Gain  Commented=on  Gain=-1
  Gain2 : Gain  Commented=on  Gain=-1
  Gain5 : Gain  Gain=10
  Gain6 : Gain  Gain=100
  Goto5 : Goto  Commented=on  GotoTag=ildmax
  Goto6 : Goto  Commented=on  GotoTag=ildmin
  Goto7 : Goto  Commented=on  GotoTag=ilqmax
  Goto8 : Goto  Commented=on  GotoTag=ilqmin
  Imax : Constant  Commented=on  Value=0.4
  Inf : Constant  Commented=on  Value=inf  OutDataTypeStr=Inherit: Inherit via back propagation
  Inf1 : Constant  Commented=on  Value=inf  OutDataTypeStr=Inherit: Inherit via back propagation
  Integrator : Integrator
  LPF : Subsystem  Commented=on
  "Lf " : Gain  Gain=Lf
  Lf1 : Gain  Gain=Lf
  One : Constant  OutDataTypeStr=Inherit: Inherit via back propagation
  One1 : Constant  Value=0.4  OutDataTypeStr=Inherit: Inherit via back propagation
  PIid : Subsystem
  PIiq : Subsystem
  PIvd : Subsystem
      settings: PortSchema="{\"entries\":[{\"content\":{\"sides\":[{\"content\":{\"connectorIds\":[\"In1\",\"In2\"]},\"type\":\"ConnectorPlacement.EquallySpacedRectSide\",\"uuid\":\"218efe14-094c-4cdd-8e62-ef6089c75bbd\"},{\"content\":{\"connectorIds\":[\"In3\",\"Out1\"],\"side\":\"RIGHT\"},\"type\":\"ConnectorPlacement.EquallySpacedRectSide\",\"uuid\":\"287e2a8a-062a-4519-a86c-f141c6982dac\"},{\"content\":{\"side\":\"TOP\"},\"type\":\"ConnectorPlacement.EquallySpacedRectSide\",\"uuid\":\"e88fce21-908c-492a-b265-04b05ce94be8\"}]},\"type\":\"ConnectorPlacement.EquallySpacedConnector\",\"uuid\":\"5c149457-da6d-4223-b1cb-56365173b759\"}],\"packageUris\":[\"http://schema.mathworks.com/mf0/Connector/R2020b\"],\"version\":\"1.0\"}"
  PIvq : Subsystem
      settings: PortSchema="{\"entries\":[{\"content\":{\"sides\":[{\"content\":{\"connectorIds\":[\"In1\",\"In2\"]},\"type\":\"ConnectorPlacement.EquallySpacedRectSide\",\"uuid\":\"5bfd4306-8421-4fdd-bae9-79740558d514\"},{\"content\":{\"connectorIds\":[\"In3\",\"Out1\"],\"side\":\"RIGHT\"},\"type\":\"ConnectorPlacement.EquallySpacedRectSide\",\"uuid\":\"1419fa8e-cc02-4da2-9592-d06db5fac946\"},{\"content\":{\"side\":\"TOP\"},\"type\":\"ConnectorPlacement.EquallySpacedRectSide\",\"uuid\":\"32aa87b6-be70-473d-807b-ed4692b27e5a\"}]},\"type\":\"ConnectorPlacement.EquallySpacedConnector\",\"uuid\":\"6bf6a9bf-c4c4-4ccc-a31e-1b4c70dd37d4\"}],\"packageUris\":[\"http://schema.mathworks.com/mf0/Connector/R2020b\"],\"version\":\"1.0\"}"
  Pmax : Constant  Commented=on  Value=0.3
  Pmax1 : Constant  Commented=on  Value=0.4
  Product{,1..3} (4 alike) : Product
  Product6 : Product  Commented=on
  RC : Subsystem  Variant=on  VariantControlMode=label  LabelModeActiveChoice=dynamic  mask{dynamic=Dynamic, R=Rcf, C=Cfi}
      mask prompts: dynamic "Dynamic behavior"; R "Parallel resistance (p.u.)"; C "Capacitance (p.u.)"
      mask init: same as VFlexP/Grid/DCAC converters/DC_VSM/VCC/dynamic_limiting/RC
      mask TypeOptions dynamic: Dynamic | Static | Static omega
  RL : Subsystem  Variant=on  VariantControlMode=label  LabelModeActiveChoice=dynamic  mask(Line){dynamic=Dynamic, R=Rf, L=Lf}
      mask prompts: dynamic "Dynamic behavior"; R "Series resistance (p.u.)"; L "Inductance (p.u.)"
      mask init: same as VFlexP/Grid/Generators/GFr/RL out
      mask Help: web('Documentation/RL.html')
      mask TypeOptions dynamic: Static | Dynamic | Static omega
  Rate Limiter : RateLimiter  SampleTimeMode=inherited
  Real-Imag to Complex : RealImagToComplex  Commented=on
  Real-Imag to Complex1 : RealImagToComplex
  Real-Imag to Complex2 : RealImagToComplex
  Real-Imag to Complex5 : RealImagToComplex
  Scope : Scope  Commented=on
      settings: ActiveDisplayYMinimum=-0.0002  ActiveDisplayYMaximum=0.00027
  Scope{1..9,11..12} (11 alike) : Scope
      Scope1 settings: ActiveDisplayYMinimum=-0.125  ActiveDisplayYMaximum=1.125  DataLoggingVariableName=ScopeData2
      Scope11 settings: ActiveDisplayYMinimum=-166.4137  ActiveDisplayYMaximum=84.6213  DataLoggingVariableName=ScopeData2
      Scope12 settings: ActiveDisplayYMinimum=-1  ActiveDisplayYMaximum=1  DataLoggingVariableName=ScopeData3
      Scope2 settings: ActiveDisplayYMinimum=-0.01117  ActiveDisplayYMaximum=0.01105  DataLoggingVariableName=ScopeData3
      Scope3 settings: ActiveDisplayYMinimum=0.77192  ActiveDisplayYMaximum=1.1413  DataLoggingVariableName=ScopeData4
      Scope4 settings: ActiveDisplayYMinimum=0.18699  ActiveDisplayYMaximum=0.31058  DataLoggingVariableName=ScopeData6
      Scope5 settings: ActiveDisplayYMinimum=-1  ActiveDisplayYMaximum=1
      Scope6 settings: ActiveDisplayYMinimum=0.11904  ActiveDisplayYMaximum=0.5824  DataLoggingVariableName=ScopeData3
      Scope7 settings: ActiveDisplayYMinimum=-1  ActiveDisplayYMaximum=1  DataLoggingVariableName=ScopeData2
      Scope8 settings: ActiveDisplayYMinimum=-1  ActiveDisplayYMaximum=1  DataLoggingVariableName=ScopeData4
      Scope9 settings: ActiveDisplayYMinimum=-5.2368  ActiveDisplayYMaximum=0.58187  DataLoggingVariableName=ScopeData2
  Scope10 : Scope  NumInputPorts=2
      settings: ActiveDisplayYMinimum=0.12846  ActiveDisplayYMaximum=0.33105
  Scope13 : Scope  NumInputPorts=2
      settings: ActiveDisplayYMinimum=-294.8154324912735  ActiveDisplayYMaximum=583.467281869242  DataLoggingVariableName=ScopeData2
  Square : Math  Operator=square
  Step : Step  Time=20  After=0.1  SampleTime=0
  Subsystem : Subsystem
  Subsystem1 : Subsystem
      settings: PortSchema="{\"entries\":[{\"content\":{\"sides\":[{\"content\":{\"connectorIds\":[\"In1\",\"In2\"]},\"type\":\"ConnectorPlacement.EquallySpacedRectSide\",\"uuid\":\"9ad25d09-f130-47a3-8a0c-c3d50f40a3f5\"},{\"content\":{\"connectorIds\":[\"Out1\",\"Out2\"],\"side\":\"RIGHT\"},\"type\":\"ConnectorPlacement.EquallySpacedRectSide\",\"uuid\":\"00c4c943-52e8-4170-9ba5-4d3b10561d7b\"},{\"content\":{\"side\":\"TOP\"},\"type\":\"ConnectorPlacement.EquallySpacedRectSide\",\"uuid\":\"98a959d8-b430-483b-8e6f-0eab01c1bae1\"},{\"content\":{\"connectorIds\":[\"In3\"],\"side\":\"BOTTOM\"},\"type\":\"ConnectorPlacement.EquallySpacedRectSide\",\"uuid\":\"01418333-d465-4764-adcc-2e5b92b6bf5d\"}]},\"type\":\"ConnectorPlacement.EquallySpacedConnector\",\"uuid\":\"e741d9d4-93b5-4bd9-8695-3e699c12860d\"}],\"packageUris\":[\"http://schema.mathworks.com/mf0/Connector/R2020b\"],\"version\":\"1.0\"}"
  Subsystem2 : Subsystem
      settings: PortSchema="{\"entries\":[{\"content\":{\"sides\":[{\"content\":{\"connectorIds\":[\"In1\",\"In2\"]},\"type\":\"ConnectorPlacement.EquallySpacedRectSide\",\"uuid\":\"9ad25d09-f130-47a3-8a0c-c3d50f40a3f5\"},{\"content\":{\"connectorIds\":[\"Out1\",\"Out2\",\"Out3\"],\"side\":\"RIGHT\"},\"type\":\"ConnectorPlacement.EquallySpacedRectSide\",\"uuid\":\"00c4c943-52e8-4170-9ba5-4d3b10561d7b\"},{\"content\":{\"side\":\"TOP\"},\"type\":\"ConnectorPlacement.EquallySpacedRectSide\",\"uuid\":\"98a959d8-b430-483b-8e6f-0eab01c1bae1\"},{\"content\":{\"connectorIds\":[\"In3\"],\"side\":\"BOTTOM\"},\"type\":\"ConnectorPlacement.EquallySpacedRectSide\",\"uuid\":\"01418333-d465-4764-adcc-2e5b92b6bf5d\"}]},\"type\":\"ConnectorPlacement.EquallySpacedConnector\",\"uuid\":\"e741d9d4-93b5-4bd9-8695-3e699c12860d\"}],\"packageUris\":[\"http://schema.mathworks.com/mf0/Connector/R2020b\"],\"version\":\"1.0\"}"
  Sum : Sum  Commented=on  Inputs=+-|
  Sum1 : Sum  Inputs=++|
  Sum11 : Sum  Inputs=|+-
  Sum{3,5..6,9,12..15} (8 alike) : Sum  Inputs=|++
  Sum2 : Sum  Inputs=-+|
  Sum4 : Sum  Inputs=++|
  Sum7 : Sum  Inputs=++|
  Sum8 : Sum  Inputs=-+|
  Switch : Switch  Commented=on  Criteria=u2 > Threshold  Threshold=1e-5  ZeroCross=off  SaturateOnIntegerOverflow=off  InputSameDT=off
  Switch1 : Switch  Commented=on  Criteria=u2 > Threshold  SaturateOnIntegerOverflow=off  InputSameDT=off
  Switch2 : Switch  Commented=on  Criteria=u2 > Threshold  SaturateOnIntegerOverflow=off  InputSameDT=off
  Switch3 : Switch  Commented=on  Criteria=u2 > Threshold  SaturateOnIntegerOverflow=off  InputSameDT=off
  VI : Subsystem  mask{L=0, R=0, Tf=0}
      mask prompts: L "Inductance (pu)"; R "Resistance (pu)"; Tf "WOF time constant (s)"
      mask init: same as VFlexP/Grid/DCAC converters/DC_VCVSC/VI
  vidref : Outport
  viqref : Outport  Port=2
  iid : Outport  Port=3
  iiq : Outport  Port=4
  vid : Outport  Port=5
  viq : Outport  Port=6
  wires:
  Product/1 -> Sum8/1
  Sum14/1 -> PIvd/1(ref)  "vodref"
  RC/2(vq) -> [voq], viqref/1, RL/4(v_out_q), Sum6/2, Scope2/1, PIvq/2(y), Cf/1  "voq"
  [omega] -> Product/2
  Lf1/1 -> Product3/2
  Sum15/1 -> PIvq/1(ref)  "voqref"
  Product3/1 -> Sum9/2
  Cf 1/1 -> Product2/2
  Cf/1 -> Product1/2
  Product1/1 -> Sum2/1
  iod/1 -> VI/1(id), Fi/1, Real-Imag to Complex5/1, RC/2(i_d_out)  "iod"
  Sum2/1 -> Sum4/2
  "Lf "/1 -> Product/1
  Sum3/1 -> Sum5/1
  [omega] -> RL/5(omega), RC/5(omega), Product3/1  "omega"
  ioq/1 -> RC/4(i_q_out), Fi2/1, VI/2(iq), Real-Imag to Complex5/2  "ioq"
  PIvd/1(Out1) -> Sum2/2
  PIvq/1(Out1) -> Scope12/1, Sum3/1
  PIid/1(Out1) -> Sum8/2
  PIiq/1(Out1) -> Sum9/1
  omega/1 -> [omega], Product2/1  "omega"
  [omega] -> Product1/1
  RL/1(id) -> RC/1(i_d_in), iid/1, Real-Imag to Complex1/1, PIid/2(y), Lf1/1, Scope10/2
  RL/2(iq) -> PIiq/2(y), "Lf "/1, iiq/1, Real-Imag to Complex1/2, RC/3(i_q_in)
  Sum8/1 -> Sum1/2  "vidref"
  Sum9/1 -> Sum6/1  "viqref"
  RC/1(vd) -> RL/2(v_out_d), Sum1/1, Scope3/1, [vod], vidref/1, PIvd/2(y), Cf 1/1
  Real-Imag to Complex5/1 -> Complex to Magnitude-Angle5/1
  Complex to Magnitude-Angle5/1 -> Scope8/1  "io_mod"
  vodref/1 -> Sum14/2  "vodref"
  voqref/1 -> Sum15/1  "voqref"
  VI/1(vd) -> Sum14/1
  VI/2(vq) -> Sum15/2
  Sum6/1 -> viq/1, [viq], RL/3(v_in_q)  "voq"
  Sum1/1 -> RL/1(v_in_d), vid/1, [vid]  "vod"
  Switch/1 -> Divide/2
  From3/1 -> LPF/1(In1)
  Constant2/1 -> Switch/3
  ? -> Goto8/1
  From4/1 -> Product6/1
  From11/1 -> Product6/2
  Product6/1 -> Sum/2
  Pmax/1 -> Sum/1
  Sum/1 -> Divide/1
  Divide/1 -> Scope/1  "ildref"
  LPF/1(Out1) -> Switch/2, Switch/1
  From12/1 -> Switch1/2, Switch2/2
  Inf1/1 -> Switch1/3, Gain1/1
  Gain1/1 -> Switch2/1
  Pmax1/1 -> Gain2/1, Switch1/1
  Gain2/1 -> Switch2/3
  Real-Imag to Complex/1 -> Complex to Magnitude-Angle/1
  Imax/1 -> Switch3/2
  Abs/1 -> Scope4/1
  Real-Imag to Complex1/1 -> Abs/1
  Sum13/1 -> Rate Limiter/1, Scope6/1, Divide1/1  "Pmax"
  One/1 -> Sum11/2
  Sum11/1 -> Dead Zone/1
  Gain6/1 -> Integrator/1
  One1/1 -> Sum13/1
  [vod] -> Divide1/2
  Sum5/1 -> Subsystem2/2(In2), Real-Imag to Complex2/2, Scope11/1
  Square/1 -> Scope7/1, Sum11/1
  Sum7/1 -> Real-Imag to Complex2/1, Subsystem2/1(In1), Scope10/1  "ildref"
  [idmax] -> Scope13/2, Sum7/1
  Gain5/1 -> Sum12/1
  Real-Imag to Complex2/1 -> Abs1/1
  Abs1/1 -> Scope5/1
  Sum12/1 -> Sum13/2
  Fi/1 -> Sum4/1
  [awp] -> PIvd/3(awp), PIvq/3(awp), Scope1/1
  Product2/1 -> Sum3/2
  Fi2/1 -> Sum5/2
  Subsystem2/1(ref) -> PIid/1(ref)
  Subsystem2/2(Out2) -> PIiq/1(ref)
  Constant/1 -> Subsystem2/3(imax)
  Subsystem2/3(awp) -> [awp]
  Sum4/1 -> Scope13/1, Sum7/2  "ildref"
  Dead Zone/1 -> [error_DC], Gain5/1, Gain6/1
  iP/1 -> [idmax]

== system VFlexP/Grid/DCAC converters/DC_VSM/VCC/static ==
  vodref : Inport
  voqref : Inport  Port=2
  iod : Inport  Port=3
  ioq : Inport  Port=4
  omega : Inport  Port=5
  Terminator : Terminator
  Terminator1 : Terminator
  Terminator2 : Terminator
  vidref : Outport
  viqref : Outport  Port=2
  wires:
  voqref/1 -> viqref/1  "voqref"
  vodref/1 -> vidref/1  "vodref"
  iod/1 -> Terminator/1  "iod"
  ioq/1 -> Terminator1/1  "ioq"
  omega/1 -> Terminator2/1  "ioq"

== system VFlexP/Grid/DCAC converters/DC_VSM/VI/WOF_d ==
  In1 : Inport
  Gain : Gain  Gain=iTf
  I : Integrator  InitialConditionSource=external  InitialCondition=Grid_op_VCVSC.op.States(6).x'
  Sum : Sum  Inputs=+-|
  Sum4 : Sum  Inputs=|+-
  Out1 : Outport
  wires:
  Sum/1 -> Out1/1
  I/1 -> Sum4/2, Sum/2
  In1/1 -> Sum4/1, Sum/1, I/2
  Sum4/1 -> Gain/1
  Gain/1 -> I/1

== system VFlexP/Grid/DCAC converters/DC_VSM/VI/WOF_q ==
  In1 : Inport
  Gain : Gain  Gain=iTf
  I : Integrator  InitialConditionSource=external  InitialCondition=Grid_op_VCVSC.op.States(7).x'
  Sum : Sum  Inputs=+-|
  Sum4 : Sum  Inputs=|+-
  Out1 : Outport
  wires:
  Sum/1 -> Out1/1
  I/1 -> Sum4/2, Sum/2
  In1/1 -> Sum4/1, Sum/1, I/2
  Sum4/1 -> Gain/1
  Gain/1 -> I/1

== system VFlexP/Grid/Generators/DFIG/Decoupling vrdqFs/Subsystem1 ==
  ird_Fs : Inport
  s : Inport  Port=2
  ws : Inport  Port=3
  ism : Inport  Port=4
  Constant : Constant
  Constant1 : Constant  Value=sigma
  Gain : Gain  Gain=Lrr_pu
  Gain2 : Gain  Gain=Lrr_pu
  Gain3 : Gain  Gain=sigma
  Product : Product  Inputs=3
  Product1 : Product
  Sum : Sum  Inputs=|++
  Sum1 : Sum  Inputs=|+-
  q : Outport
  wires:
  Product/1 -> q/1
  ird_Fs/1 -> Gain2/1
  ws/1 -> Product/2
  Product1/1 -> Sum/2
  s/1 -> Product/1
  Gain/1 -> Product1/1
  Gain2/1 -> Gain3/1
  Gain3/1 -> Sum/1
  Constant/1 -> Sum1/1
  Constant1/1 -> Sum1/2
  Sum1/1 -> Gain/1
  ism/1 -> Product1/2
  Sum/1 -> Product/3

== system VFlexP/Grid/Generators/DFIG/Decoupling vrdqFs/Subsystem2 ==
  irq_Fs : Inport
  s : Inport  Port=2
  ws : Inport  Port=3
  Constant : Constant  Value=sigma
  Display : Display
  Gain : Gain  Gain=Lrr_pu
  Gain1 : Gain  Gain=sigma
  Product : Product
  Product1 : Product
  d : Outport
  wires:
  Gain/1 -> Gain1/1
  Product/1 -> Gain/1
  s/1 -> Product/1
  Gain1/1 -> Product1/2
  ws/1 -> Product/2
  irq_Fs/1 -> Product1/1
  Product1/1 -> d/1
  Constant/1 -> Display/1
